simulink model "fen_models"  (Simulink 7.9)
settings: Solver=ode45  StartTime=0.0  StopTime=1000  RelTol=1e-3
undefined symbols (not defined in the file): beta, c1, c2, h_high_cm, h_low_cm, h_mid_cm, k1_high, k1_low, k1_mid, k2_high, k2_low, k2_mid, u_high, u_low, u_mid
libraries: simulink x3
settings Model: Creator=matias  LastModifiedBy=matias
settings DebuggingCC: SolverPrmCheckMsg=none

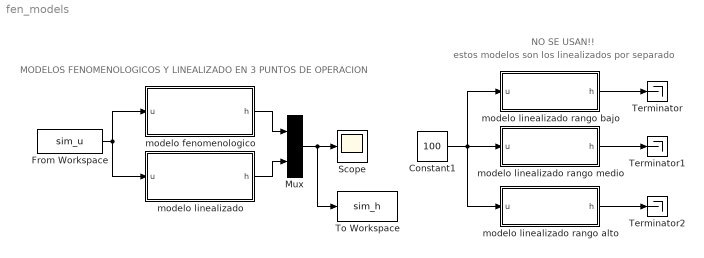
== system fen_models ==
  note: estos modelos son los linealizados por separado
  note: NO SE USAN!!
  note: MODELOS FENOMENOLOGICOS
      | Y LINEALIZADO EN 3 PUNTOS DE OPERACION
  Constant1 : Constant  Value=100
  From Workspace : FromWorkspace  VariableName=sim_u  SampleTime=0
  Mux : Mux  Inputs=2
  Scope : Scope
      settings: TimeRange=1200  YMin=0  YMax=100
  Terminator : Terminator
  Terminator1 : Terminator
  Terminator2 : Terminator
  To Workspace : ToWorkspace  VariableName=sim_h  SampleTime=-1  SaveFormat=Timeseries
  modelo fenomenologico : Subsystem  Tag=Modelo Fenomenologico
  modelo linealizado : Subsystem  Tag=Modelo Fenomenologico
  modelo linealizado rango alto : Subsystem
  modelo linealizado rango bajo : Subsystem
  modelo linealizado rango medio : Subsystem
  wires:
  From Workspace/1 -> modelo fenomenologico/1(u), modelo linealizado/1(u)
  Mux/1 -> Scope/1, To Workspace/1
  modelo fenomenologico/1(h) -> Mux/1
  modelo linealizado/1(h) -> Mux/2
  modelo linealizado rango bajo/1(h) -> Terminator/1
  modelo linealizado rango medio/1(h) -> Terminator1/1
  modelo linealizado rango alto/1(h) -> Terminator2/1
  Constant1/1 -> modelo linealizado rango medio/1(u), modelo linealizado rango bajo/1(u), modelo linealizado rango alto/1(u)

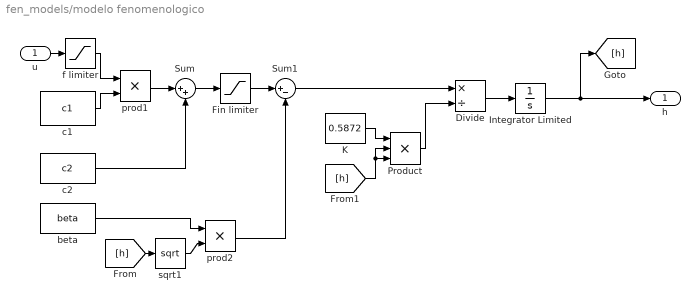
== system fen_models/modelo fenomenologico ==
  u : Inport
  Divide : Product  Inputs=*/
  Fin limiter : Saturate  UpperLimit=inf  LowerLimit=0
  Integrator Limited : Integrator  InitialCondition=0.1  LimitOutput=on  UpperSaturationLimit=80  LowerSaturationLimit=0.1
  K : Constant  Value=0.5872
  Product : Product  Inputs=3  RndMeth=Zero
  Sum : Sum  Inputs=|++
  Sum1 : Sum  Inputs=|+-
  beta : Constant  Value=beta
  c1 : Constant  Value=c1
  c2 : Constant  Value=c2
  f limiter : Saturate  UpperLimit=100  LowerLimit=0
  prod1 : Product  RndMeth=Zero
  prod2 : Product  RndMeth=Zero
  sqrt1 : Sqrt  SaturateOnIntegerOverflow=on
  h : Outport
  wires:
  f limiter/1 -> prod1/1
  c1/1 -> prod1/2
  prod1/1 -> Sum/1
  c2/1 -> Sum/2
  beta/1 -> prod2/1
  prod2/1 -> Sum1/2
  sqrt1/1 -> prod2/2
  Sum1/1 -> Divide/1
  [h] -> sqrt1/1
  Product/1 -> Divide/2
  K/1 -> Product/1
  [h] -> Product/2, Product/3
  Divide/1 -> Integrator Limited/1
  Integrator Limited/1 -> h/1, [h]
  Sum/1 -> Fin limiter/1
  Fin limiter/1 -> Sum1/1
  u/1 -> f limiter/1

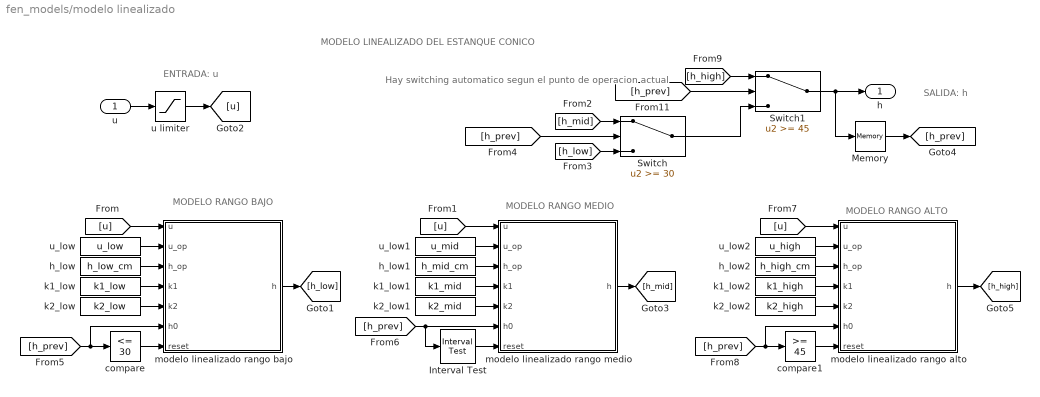
== system fen_models/modelo linealizado ==
  note: MODELO RANGO BAJO
  note: MODELO RANGO MEDIO
  note: MODELO RANGO ALTO
  note: ENTRADA: u
  note: MODELO LINEALIZADO DEL ESTANQUE CONICO
  note: Hay switching automatico segun
      | el punto de operacion actual
  note: SALIDA: h
  u : Inport
  Interval Test : simulink/Logic and Bit Operations/Interval Test  IntervalClosedRight=on  uplimit=45  IntervalClosedLeft=on  lowlimit=30  OutDataTypeStr=boolean
  Memory : Memory
  Switch : Switch  Threshold=30
  Switch1 : Switch  Threshold=45
  compare : simulink/Logic and Bit Operations/Compare To Constant  relop=<=  const=30  OutDataTypeStr=boolean
  compare1 : simulink/Logic and Bit Operations/Compare To Constant  relop=>=  const=45  OutDataTypeStr=boolean
  h_low : Constant  Value=h_low_cm
  h_low1 : Constant  Value=h_mid_cm
  h_low2 : Constant  Value=h_high_cm
  k1_low : Constant  Value=k1_low
  k1_low1 : Constant  Value=k1_mid
  k1_low2 : Constant  Value=k1_high
  k2_low : Constant  Value=k2_low
  k2_low1 : Constant  Value=k2_mid
  k2_low2 : Constant  Value=k2_high
  modelo linealizado rango alto : Subsystem
  modelo linealizado rango bajo : Subsystem
  modelo linealizado rango medio : Subsystem
  u limiter : Saturate  UpperLimit=100  LowerLimit=0
  u_low : Constant  Value=u_low
  u_low1 : Constant  Value=u_mid
  u_low2 : Constant  Value=u_high
  h : Outport
  wires:
  u/1 -> u limiter/1
  u_low/1 -> modelo linealizado rango bajo/2(u_op)
  h_low/1 -> modelo linealizado rango bajo/3(h_op)
  k1_low/1 -> modelo linealizado rango bajo/4(k1)
  k2_low/1 -> modelo linealizado rango bajo/5(k2)
  modelo linealizado rango bajo/1(h) -> [h_low]
  u limiter/1 -> [u]
  [u] -> modelo linealizado rango bajo/1(u)
  u_low1/1 -> modelo linealizado rango medio/2(u_op)
  h_low1/1 -> modelo linealizado rango medio/3(h_op)
  k1_low1/1 -> modelo linealizado rango medio/4(k1)
  k2_low1/1 -> modelo linealizado rango medio/5(k2)
  modelo linealizado rango medio/1(h) -> [h_mid]
  [u] -> modelo linealizado rango medio/1(u)
  [h_mid] -> Switch/1
  [h_low] -> Switch/3
  Memory/1 -> [h_prev]
  [h_prev] -> Switch/2
  [h_prev] -> compare/1, modelo linealizado rango bajo/6(h0)
  compare/1 -> modelo linealizado rango bajo/7(reset)
  [h_prev] -> modelo linealizado rango medio/6(h0), Interval Test/1
  Interval Test/1 -> modelo linealizado rango medio/7(reset)
  u_low2/1 -> modelo linealizado rango alto/2(u_op)
  h_low2/1 -> modelo linealizado rango alto/3(h_op)
  k1_low2/1 -> modelo linealizado rango alto/4(k1)
  k2_low2/1 -> modelo linealizado rango alto/5(k2)
  modelo linealizado rango alto/1(h) -> [h_high]
  [u] -> modelo linealizado rango alto/1(u)
  [h_prev] -> compare1/1, modelo linealizado rango alto/6(h0)
  compare1/1 -> modelo linealizado rango alto/7(reset)
  [h_high] -> Switch1/1
  Switch/1 -> Switch1/3
  [h_prev] -> Switch1/2
  Switch1/1 -> h/1, Memory/1

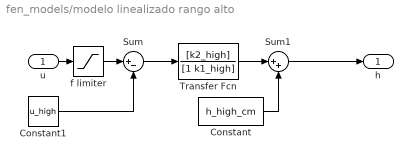
== system fen_models/modelo linealizado rango alto ==
  u : Inport
  Constant : Constant  Value=h_high_cm
  Constant1 : Constant  Value=u_high
  Sum : Sum  Inputs=|+-
  Sum1 : Sum  Inputs=|++
  Transfer Fcn : TransferFcn  Numerator=[k2_high]  Denominator=[1 k1_high]
  f limiter : Saturate  UpperLimit=100  LowerLimit=0
  h : Outport
  wires:
  Constant1/1 -> Sum/2
  Sum1/1 -> h/1
  Constant/1 -> Sum1/2
  f limiter/1 -> Sum/1
  u/1 -> f limiter/1
  Sum/1 -> Transfer Fcn/1
  Transfer Fcn/1 -> Sum1/1

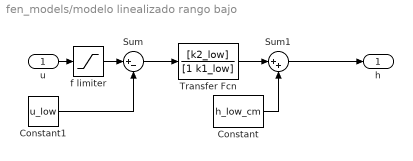
== system fen_models/modelo linealizado rango bajo ==
  u : Inport
  Constant : Constant  Value=h_low_cm
  Constant1 : Constant  Value=u_low
  Sum : Sum  Inputs=|+-
  Sum1 : Sum  Inputs=|++
  Transfer Fcn : TransferFcn  Numerator=[k2_low]  Denominator=[1 k1_low]
  f limiter : Saturate  UpperLimit=100  LowerLimit=0
  h : Outport
  wires:
  Constant1/1 -> Sum/2
  Sum1/1 -> h/1
  Constant/1 -> Sum1/2
  f limiter/1 -> Sum/1
  u/1 -> f limiter/1
  Sum/1 -> Transfer Fcn/1
  Transfer Fcn/1 -> Sum1/1

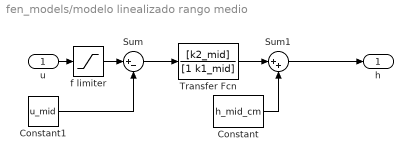
== system fen_models/modelo linealizado rango medio ==
  u : Inport
  Constant : Constant  Value=h_mid_cm
  Constant1 : Constant  Value=u_mid
  Sum : Sum  Inputs=|+-
  Sum1 : Sum  Inputs=|++
  Transfer Fcn : TransferFcn  Numerator=[k2_mid]  Denominator=[1 k1_mid]
  f limiter : Saturate  UpperLimit=100  LowerLimit=0
  h : Outport
  wires:
  Constant1/1 -> Sum/2
  Sum1/1 -> h/1
  Constant/1 -> Sum1/2
  f limiter/1 -> Sum/1
  u/1 -> f limiter/1
  Sum/1 -> Transfer Fcn/1
  Transfer Fcn/1 -> Sum1/1

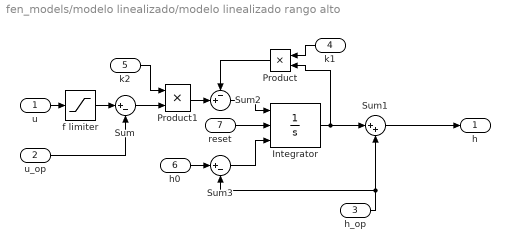
== system fen_models/modelo linealizado/modelo linealizado rango alto ==
  u : Inport
  u_op : Inport  Port=2
  h_op : Inport  Port=3
  k1 : Inport  Port=4
  k2 : Inport  Port=5
  h0 : Inport  Port=6
  reset : Inport  Port=7
  Integrator : Integrator  ExternalReset=rising  InitialConditionSource=external
  Product : Product  RndMeth=Zero
  Product1 : Product  RndMeth=Zero
  Sum : Sum  Inputs=|+-
  Sum1 : Sum  Inputs=|++
  Sum2 : Sum  Inputs=-+|
  Sum3 : Sum  Inputs=|+-
  f limiter : Saturate  UpperLimit=100  LowerLimit=0
  h : Outport
  wires:
  u_op/1 -> Sum/2
  Integrator/1 -> Sum1/1, Product/2
  Sum1/1 -> h/1
  h_op/1 -> Sum1/2, Sum3/2
  f limiter/1 -> Sum/1
  u/1 -> f limiter/1
  Sum2/1 -> Integrator/1
  Product1/1 -> Sum2/2
  Product/1 -> Sum2/1
  reset/1 -> Integrator/2
  h0/1 -> Sum3/1
  Sum3/1 -> Integrator/3
  k1/1 -> Product/1
  Sum/1 -> Product1/2
  k2/1 -> Product1/1

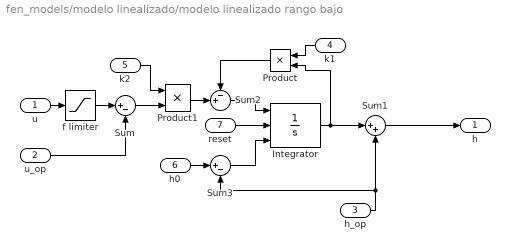
== system fen_models/modelo linealizado/modelo linealizado rango bajo ==
  u : Inport
  u_op : Inport  Port=2
  h_op : Inport  Port=3
  k1 : Inport  Port=4
  k2 : Inport  Port=5
  h0 : Inport  Port=6
  reset : Inport  Port=7
  Integrator : Integrator  ExternalReset=rising  InitialConditionSource=external
  Product : Product  RndMeth=Zero
  Product1 : Product  RndMeth=Zero
  Sum : Sum  Inputs=|+-
  Sum1 : Sum  Inputs=|++
  Sum2 : Sum  Inputs=-+|
  Sum3 : Sum  Inputs=|+-
  f limiter : Saturate  UpperLimit=100  LowerLimit=0
  h : Outport
  wires:
  u_op/1 -> Sum/2
  Integrator/1 -> Sum1/1, Product/2
  Sum1/1 -> h/1
  h_op/1 -> Sum1/2, Sum3/2
  f limiter/1 -> Sum/1
  u/1 -> f limiter/1
  Sum2/1 -> Integrator/1
  Product1/1 -> Sum2/2
  Product/1 -> Sum2/1
  reset/1 -> Integrator/2
  h0/1 -> Sum3/1
  Sum3/1 -> Integrator/3
  k1/1 -> Product/1
  Sum/1 -> Product1/2
  k2/1 -> Product1/1

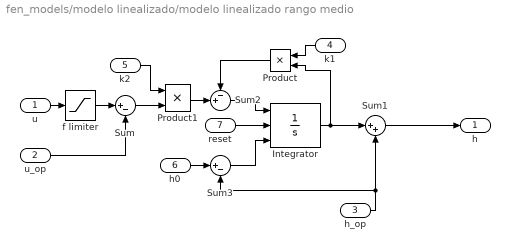
== system fen_models/modelo linealizado/modelo linealizado rango medio ==
  u : Inport
  u_op : Inport  Port=2
  h_op : Inport  Port=3
  k1 : Inport  Port=4
  k2 : Inport  Port=5
  h0 : Inport  Port=6
  reset : Inport  Port=7
  Integrator : Integrator  ExternalReset=rising  InitialConditionSource=external
  Product : Product  RndMeth=Zero
  Product1 : Product  RndMeth=Zero
  Sum : Sum  Inputs=|+-
  Sum1 : Sum  Inputs=|++
  Sum2 : Sum  Inputs=-+|
  Sum3 : Sum  Inputs=|+-
  f limiter : Saturate  UpperLimit=100  LowerLimit=0
  h : Outport
  wires:
  u_op/1 -> Sum/2
  Integrator/1 -> Sum1/1, Product/2
  Sum1/1 -> h/1
  h_op/1 -> Sum1/2, Sum3/2
  f limiter/1 -> Sum/1
  u/1 -> f limiter/1
  Sum2/1 -> Integrator/1
  Product1/1 -> Sum2/2
  Product/1 -> Sum2/1
  reset/1 -> Integrator/2
  h0/1 -> Sum3/1
  Sum3/1 -> Integrator/3
  k1/1 -> Product/1
  Sum/1 -> Product1/2
  k2/1 -> Product1/1
